simulink model "Leg_4DOF"  (Simulink 8.9)
settings: Solver=VariableStepAuto  StartTime=0.0  StopTime=50  MaxStep=1e-2  RelTol=1e-3  EnableMultiTasking=on
values from neighbouring files (symbols this model uses):
  beta = 10    [Copy_of_Init_4DOF.m]
  BodyContact = [ 4 4 ]    [Copy_of_Init_4DOF.m]
  BodyContactPositions = [ contact_point_h, contact_point_t ]    [Copy_of_Init_4DOF.m]
  dqInit = [ 0 0 0 0 ]'    [Copy_of_Init_4DOF.m]
  G = g*ez    [Copy_of_Init_4DOF.m]
  G_ctrl = g*ez    [Copy_of_Init_4DOF.m]
  h = [ ez -ey -ey -ey ]    [Copy_of_Init_4DOF.m]
  h_ctrl = [ ez -ey -ey -ey ]    [Copy_of_Init_4DOF.m]
  Inertia = [ I_base I_hip I_thigh I_shin I_foot ]    [Copy_of_Init_4DOF.m]
  Inertia_ctrl = [ I_base I_hip I_thigh I_shin I_foot ]    [Copy_of_Init_4DOF.m]
  joint_type = [ 1 0 0 0 ]    [Copy_of_Init_4DOF.m]
  k_b = 10    [Copy_of_Init_4DOF.m]
  Kd = kd*eye(n)    [Copy_of_Init_4DOF.m]
  Ki = ki*eye(n)    [Copy_of_Init_4DOF.m]
  Kp = kp*eye(n)    [Copy_of_Init_4DOF.m]
  L = [ l_base_hip l_hip_thigh l_thigh_shin l_shin_foot ]    [Copy_of_Init_4DOF.m]
  L_ctrl = [ l_base_hip l_hip_thigh l_thigh_shin l_shin_foot ]    [Copy_of_Init_4DOF.m]
  Mass = [ mass_base mass_hip mass_thigh mass_shin mass_foot ]    [Copy_of_Init_4DOF.m]
  Mass_ctrl = [ mass_base mass_hip mass_thigh mass_shin mass_foot ]    [Copy_of_Init_4DOF.m]
  n = 4    [Copy_of_Init_4DOF.m]
  offset = zeros(n,1)    [Copy_of_Init_4DOF.m]
  qInit = [ 0 pi/2 -pi/2 0 ]'    [Copy_of_Init_4DOF.m]
  R = [ r_base r_hip r_thigh r_shin r_foot ]    [Copy_of_Init_4DOF.m]
  R_ctrl = [ r_base r_hip r_thigh r_shin r_foot ]    [Copy_of_Init_4DOF.m]
  s_z = 2    [Copy_of_Init_4DOF.m]
  w = [ 0   ; 0.5*pi*ones(3,1) ]    [Copy_of_Init_4DOF.m]
undefined symbols (not defined in the file or in its folder): A, Fstate0
libraries: simulink x1
settings Model: Creator=Ultron  LastModifiedBy=Ultron
settings DataIOCC: SignalLoggingSaveFormat=Dataset
settings DebuggingCC: UnderspecifiedInitializationDetection=Simplified  MergeDetectMultiDrivingBlocksExec=error  FcnCallInpInsideContextMsg=error  StateNameClashWarn=none
settings GRTTargetCC: CombineOutputUpdateFcns=on  GRTInterface=off

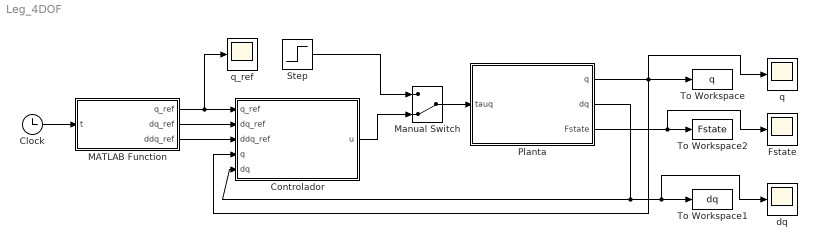
== system Leg_4DOF ==
  Clock : Clock
  Controlador : Subsystem
  Fstate : Scope
  MATLAB Function : MATLAB Function  TreatAsAtomicUnit=on
  Manual Switch : ManualSwitch  CurrentSetting=0
  Planta : Subsystem
  Step : Step  Before=[0;0;0;0]  After=[1;1;1;1]  SampleTime=0
  To Workspace : ToWorkspace  VariableName=q  SaveFormat=Timeseries  SampleTime=-1
  To Workspace1 : ToWorkspace  VariableName=dq  SaveFormat=Timeseries  SampleTime=-1
  To Workspace2 : ToWorkspace  VariableName=Fstate  SaveFormat=Timeseries  SampleTime=-1
  dq : Scope
  q : Scope
  q_ref : Scope
  wires:
  Planta/2(dq) -> dq/1, To Workspace1/1, Controlador/5(dq)
  Manual Switch/1 -> Planta/1(tauq)
  Step/1 -> Manual Switch/1
  Controlador/1(u) -> Manual Switch/2
  MATLAB Function/1(q_ref) -> q_ref/1, Controlador/1(q_ref)
  MATLAB Function/2(dq_ref) -> Controlador/2(dq_ref)
  MATLAB Function/3(ddq_ref) -> Controlador/3(ddq_ref)
  Clock/1 -> MATLAB Function/1(t)
  Planta/1(q) -> Controlador/4(q), To Workspace/1, q/1
  Planta/3(Fstate) -> Fstate/1, To Workspace2/1

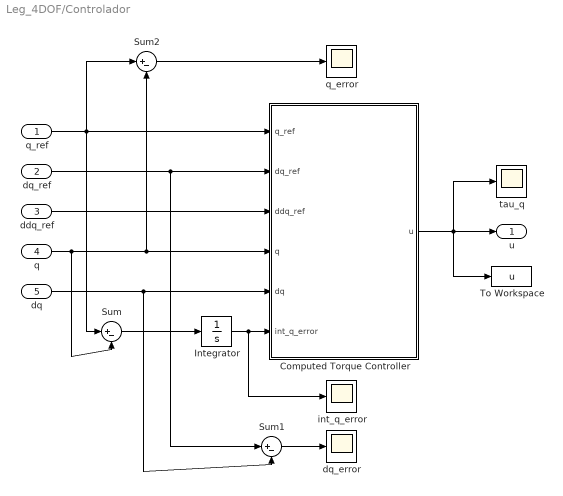
== system Leg_4DOF/Controlador ==
  q_ref : Inport
  dq_ref : Inport  Port=2
  ddq_ref : Inport  Port=3
  q : Inport  Port=4
  dq : Inport  Port=5
  Computed Torque Controller : MATLAB Function  TreatAsAtomicUnit=on
  Integrator : Integrator  InitialCondition=zeros(4,1)
  Sum : Sum  Inputs=|+-
  Sum1 : Sum  Inputs=|+-
  Sum2 : Sum  Inputs=|+-
  To Workspace : ToWorkspace  VariableName=u  SaveFormat=Timeseries  SampleTime=-1
  dq_error : Scope
  int_q_error : Scope
  q_error : Scope
  tau_q : Scope
  u : Outport
  wires:
  Computed Torque Controller/1(u) -> To Workspace/1, tau_q/1, u/1
  q_ref/1 -> Sum2/1, Sum/1, Computed Torque Controller/1(q_ref)
  dq_ref/1 -> Sum1/1, Computed Torque Controller/2(dq_ref)
  q/1 -> Sum/2, Computed Torque Controller/4(q), Sum2/2
  Sum1/1 -> dq_error/1
  ddq_ref/1 -> Computed Torque Controller/3(ddq_ref)
  dq/1 -> Sum1/2, Computed Torque Controller/5(dq)
  Sum/1 -> Integrator/1
  Integrator/1 -> int_q_error/1, Computed Torque Controller/6(int_q_error)
  Sum2/1 -> q_error/1

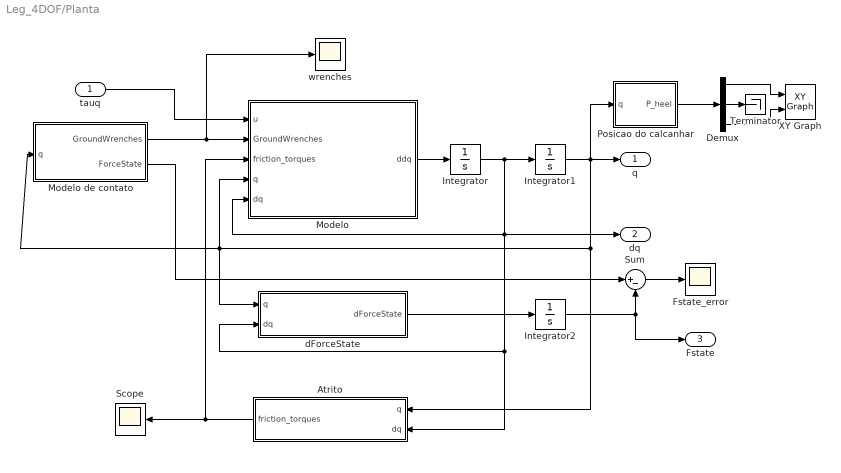
== system Leg_4DOF/Planta ==
  tauq : Inport
  Atrito : MATLAB Function  TreatAsAtomicUnit=on
  Demux : Demux  Outputs=3
  Fstate_error : Scope
  Integrator : Integrator  InitialCondition=dqInit
  Integrator1 : Integrator  InitialCondition=qInit
  Integrator2 : Integrator  InitialCondition=Fstate0
  Modelo : MATLAB Function  TreatAsAtomicUnit=on
  Modelo de contato : MATLAB Function  TreatAsAtomicUnit=on
  Posicao do calcanhar : MATLAB Function  TreatAsAtomicUnit=on
  Scope : Scope
  Sum : Sum  Inputs=|+-
  Terminator : Terminator
  XY Graph : simulink/Sinks/XY Graph  xmin=-2  xmax=2  ymin=-2  ymax=2  st=-1
  dForceState : MATLAB Function  TreatAsAtomicUnit=on
  wrenches : Scope
  q : Outport
  dq : Outport  Port=2
  Fstate : Outport  Port=3
  wires:
  Integrator1/1 -> dForceState/1(q), Modelo de contato/1(q), Modelo/4(q), Atrito/1(q), Posicao do calcanhar/1(q), q/1
  Modelo/1(ddq) -> Integrator/1
  Integrator/1 -> Integrator1/1, Modelo/5(dq), dForceState/2(dq), Atrito/2(dq), dq/1
  Atrito/1(friction_torques) -> Modelo/3(friction_torques), Scope/1
  tauq/1 -> Modelo/1(u)
  Modelo de contato/1(GroundWrenches) -> wrenches/1, Modelo/2(GroundWrenches)
  Posicao do calcanhar/1(P_heel) -> Demux/1
  Demux/2 -> Terminator/1
  Demux/1 -> XY Graph/1
  Demux/3 -> XY Graph/2
  Integrator2/1 -> Sum/2, Fstate/1
  dForceState/1(dForceState) -> Integrator2/1
  Modelo de contato/2(ForceState) -> Sum/1
  Sum/1 -> Fstate_error/1

== matlab function Controlador/Computed Torque Controller ==
  data: q_ref input double; dq_ref input double; ddq_ref input double; u output double; q input double; dq input double; int_q_error input double; joint_type parameter double; Mass_ctrl parameter double; Inertia_ctrl parameter double; R_ctrl parameter double; L_ctrl parameter double; h_ctrl parameter double; G_ctrl parameter double; Kp parameter double; Kd parameter double; Ki parameter double
function u = fcn(q_ref, dq_ref, ddq_ref, q, dq, int_q_error, joint_type, Mass_ctrl, Inertia_ctrl, R_ctrl, L_ctrl, h_ctrl, G_ctrl, Kp, Kd, Ki )
%% Prostectics control

v = ddq_ref + Kd*(dq_ref - dq) + Kp*(q_ref - q) + Ki*int_q_error;
u = prosthetics_inverse_dynamics( q, dq, v, joint_type, Mass_ctrl, Inertia_ctrl, R_ctrl, L_ctrl, h_ctrl, G_ctrl );

== matlab function Planta/Modelo ==
  data: u input double; GroundWrenches input double; friction_torques input double; q input double; dq input double; joint_type parameter double; Mass parameter double; Inertia parameter double; R parameter double; L parameter double; h parameter double; G parameter double; ddq output double; BodyContactPositions parameter double; BodyContact parameter double
function ddq = fcn( u, GroundWrenches, friction_torques, q, dq, joint_type, Mass, Inertia, R, L, h, G, BodyContactPositions,  BodyContact )
% direct dynamics

% n = length(q);

% coder.extrinsic('model_prosthetics_mex');
% ddq = coder.nullcopy(zeros(n,1));
% Friction_torques = coder.nullcopy(zeros(n,1));

ddq = model_prosthetics( u, q, dq, joint_type, Mass, Inertia, R, L, h, G, friction_torques, BodyContact, GroundWrenches, BodyContactPositions );
% ddq = model_prosthetics_mex( u, q, dq, joint_type, Mass, Inertia, R, L, h, G, friction_coefs, BodyContact, BodyContactWrenches, BodyContactPositions );

== matlab function MATLAB Function ==
  data: t input double; q_ref output double; dq_ref output double; ddq_ref output double; n parameter double; A parameter double; offset parameter double; w parameter double
function [ q_ref, dq_ref, ddq_ref ] = fcn( t, n,  A, offset, w)
% generate reference

q_ref = A*sin(w*t + offset);
dq_ref = A*w*cos(w*t + offset);
ddq_ref = -A*(w^2)*sin(w*t + offset);

% q_ref = zeros(n,1);
% dq_ref = zeros(n,1);
% ddq_ref = zeros(n,1);
% 
% for i = 1:n
%     q_ref(i) = A(i)*sin(w(i)*t + offset(i));
%     dq_ref(i) = A(i)*w(i)*cos(w(i)*t + offset(i));
%     ddq_ref(i) = -A(i)*(w(i)^2)*sin(w(i)*t + offset(i));
% end

== matlab function Planta/Atrito ==
  data: friction_torques output double; q input double; dq input double
function friction_torques = fcn( q, dq )
%% Joint friction model
n = length(q);
friction_torques = zeros(n,1);

== matlab function Planta/Posicao do calcanhar ==
  data: q input double; P_heel output double; joint_type parameter double; h parameter double; L parameter double
function P_heel = fcn( q, joint_type,  h, L)
%% Cinematica direta do pe

point = zeros(3,1);

P_heel = prosthetics_forward_kinematics( q, L, h, 4, point, joint_type );

== matlab function Planta/Modelo de contato ==
  data: GroundWrenches output double; q input double; BodyContactPositions parameter double; s_z parameter double; L parameter double; h parameter double; beta parameter double; k_b parameter double; joint_type parameter double; ForceState output double
function [ GroundWrenches, ForceState ] = fcn( q, BodyContactPositions, s_z, L, h, beta,  k_b, joint_type )
% function BodyContactWrenches = fcn( t, q, L, h, BodyContactPositions, joint_type, sz, beta, kb)
% Esta função calcula as forças de contato com o chão

[ GroundWrenches, ForceState ] = ground_model( q, BodyContactPositions, s_z, L, h, beta,  k_b, joint_type );

== matlab function Planta/dForceState ==
  data: q input double; dq input double; dForceState output double; L parameter double; h parameter double; joint_type parameter double; BodyContactPositions parameter double; s_z parameter double; beta parameter double; k_b parameter double
function dForceState = fcn( q, dq, L, h, joint_type,  BodyContactPositions, s_z, beta, k_b)
%% Dinâmica do modelo de contato (em coordenadas inerciais)

%% Computes the velocity body twist of the given point.
body = 4;
contact_point_h = BodyContactPositions(:,1);
contact_point_t = BodyContactPositions(:,2);
V_h = prosthetics_diff_kinematics( q, dq, L, h, body, contact_point_h, joint_type );
V_t = prosthetics_diff_kinematics( q, dq, L, h, body, contact_point_t, joint_type );

%% Computes 
[ P_h, R_h ] = prosthetics_forward_kinematics( q, L, h, body, contact_point_h, joint_type );
[ P_t, R_t ] = prosthetics_forward_kinematics( q, L, h, body, contact_point_h, joint_type );
z_h = P_h(3);
z_t = P_t(3);

%% Converts body linear velocity into inertial velocty
v_h = R_h*V_h(1:3);
v_t = R_t*V_t(1:3);

dz_h = v_h(3);
dz_t = v_t(3);

dF_zh = -(k_b/2)*dz_h*(1+sign(z_h - s_z));
dF_zt = -(k_b/2)*dz_t*(1+sign(z_t - s_z));

dF_xh = beta*dF_zh;
dF_xt = beta*dF_zt;

dForceState = [ dF_zh dF_zt dF_xh dF_xt ]';
